simulink model "Modeling_of_Wind_Turbine"  (R2023a)
settings: Solver=VariableStepAuto  StartTime=0.0  StopTime=10.0  RelTol=1e-3
settings Model: Creator=SAHIL FADNAVIS  LastModifiedBy=SAHIL FADNAVIS

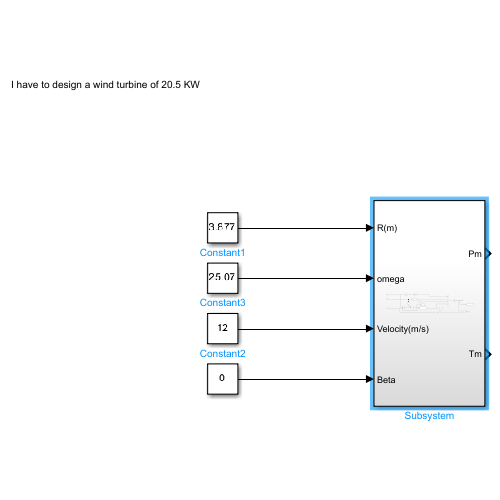
[thumbnail: Simulink's stored preview of the top-level diagram]
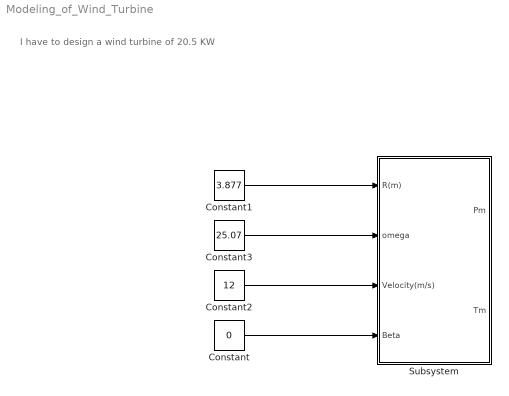
== system Modeling_of_Wind_Turbine ==
  note: I have to design a wind turbine of 20.5 KW
  Constant : Constant  Value=0
  Constant1 : Constant  Value=3.877
  Constant2 : Constant  Value=12
  Constant3 : Constant  Value=25.07
  Subsystem : Subsystem
  wires:
  Constant/1 -> Subsystem/4(Beta)
  Constant3/1 -> Subsystem/2(omega)
  Constant1/1 -> Subsystem/1(R(m))
  Constant2/1 -> Subsystem/3(Velocity(m/s))

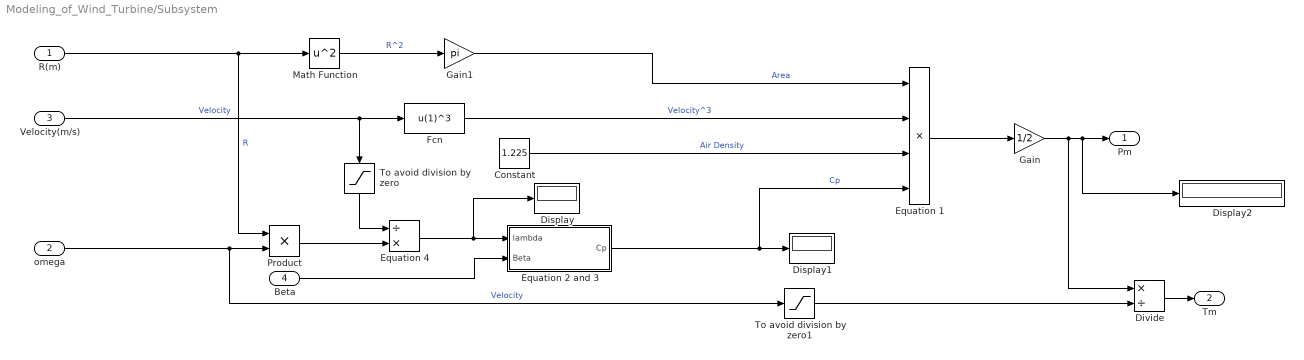
== system Modeling_of_Wind_Turbine/Subsystem ==
  R(m) : Inport
  omega : Inport  Port=2
  Velocity(m/s) : Inport  Port=3
  Beta : Inport  Port=4
  Constant : Constant  Value=1.225
  Display : Display
  Display1 : Display
  Display2 : Display
      settings: Format=decimal (Stored Integer)
  Divide : Product  Inputs=*/
  Equation 1 : Product  Inputs=4
  Equation 2 and 3 : Subsystem
  Equation 4 : Product  Inputs=/*
  Fcn : Fcn  Expr=u(1)^3
  Gain : Gain  Gain=1/2
  Gain1 : Gain  Gain=pi
  Math Function : Math  Operator=square
  Product : Product
  To avoid division by zero : Saturate  UpperLimit=inf  LowerLimit=1e-6
  To avoid division by zero1 : Saturate  UpperLimit=1e6  LowerLimit=1e-6
  Pm : Outport
  Tm : Outport  Port=2
  wires:
  Gain/1 -> Divide/1, Display2/1, Pm/1
  Equation 1/1 -> Gain/1
  Gain1/1 -> Equation 1/1  "Area"
  Fcn/1 -> Equation 1/2  "Velocity^3"
  Constant/1 -> Equation 1/3  "Air Density"
  Equation 2 and 3/1(Cp) -> Display1/1, Equation 1/4  "Cp"
  R(m)/1 -> Product/1, Math Function/1  "R"
  Math Function/1 -> Gain1/1  "R^2"
  Velocity(m/s)/1 -> Fcn/1, To avoid division by zero/1  "Velocity"
  omega/1 -> To avoid division by zero1/1, Product/2  "Velocity"
  Equation 4/1 -> Display/1, Equation 2 and 3/1(lambda)
  Beta/1 -> Equation 2 and 3/2(Beta)
  Product/1 -> Equation 4/2
  To avoid division by zero/1 -> Equation 4/1
  Divide/1 -> Tm/1
  To avoid division by zero1/1 -> Divide/2

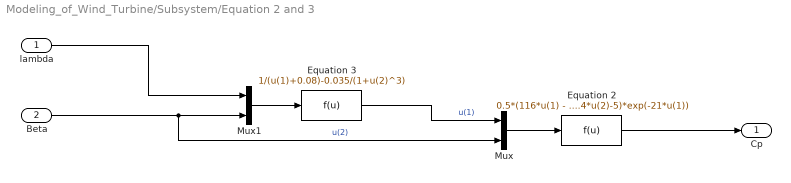
== system Modeling_of_Wind_Turbine/Subsystem/Equation 2 and 3 ==
  lambda : Inport
  Beta : Inport  Port=2
  Equation 2 : Fcn  Expr=0.5*(116*u(1) - 0.4*u(2)-5)*exp(-21*u(1))
  Equation 3 : Fcn  Expr=1/(u(1)+0.08)-0.035/(1+u(2)^3)
  Mux : Mux  Inputs=2
  Mux1 : Mux  Inputs=2
  Cp : Outport
  wires:
  Equation 2/1 -> Cp/1
  Equation 3/1 -> Mux/1  "u(1)"
  Beta/1 -> Mux/2, Mux1/2  "u(2)"
  Mux1/1 -> Equation 3/1
  Mux/1 -> Equation 2/1
  lambda/1 -> Mux1/1
